simulink model "lead_acid_battery_estim"  (R2014a)
settings: Solver=ode15s  StartTime=0.0  StopTime=14787  RelTol=1e-3
PreLoadFcn:
  | ssc_lead_acid_battery_ini
  | load Measured_DATA
PostLoadFcn:
  | open_system([bdroot '/Orig. Values']);
  | warning off Simulink:blocks:MatchingFromNotFound
  | warning off Simulink:Engine:MdlFileShadowedByFile
undefined symbols (not defined in the file): Kt, Kt_Temps, sigbuilder_block, theta_f, theta_init
libraries: fl_lib x15, nesl_utility x6, LeadAcidBattery_lib x6
Description:
  | Lead-acid battery
  | 
  | This demo implements a model of a lead-acid battery cell using the Simscape
  | language to implement the nonlinear equations of the equivalent circuit
  | components. In this way, as opposed to modeling entirely in Simulink, the
  | connection between model components and the defining physical equations is
  | more easily understood. For the defining equations and their validation,
  | see Jackey, R. "A Simple, Effective Lead-Acid Battery Modeling Process for
  | Electrical System Component Selection",  SAE World Congress & Exhibition,
  | April 2007, ref. 2007-01-0778.
  | 
  | In this simulation, initially the battery is discharged at a constant current of 10A.
  | The battery is then recharged at a constant 10A back to the initial state of
  | charge. A simple thermal model is used to model battery temperature. It is
  | assumed that cooling is primarily via convection, and that heating is primarily
  | from battery internal resistance, R2. A standard 12 V lead-acid battery can
  | be modeled by connecting six copies of the 2V battery cell block in series.
  | Copyright 2014 The MathWorks, Inc.
settings Model: Creator=rhyde  LastModifiedBy=psanghvi
settings DataIOCC: ExternalInput=[Input_time, Input_Current_DATA]  LoadExternalInput=on  SignalLoggingSaveFormat=ModelDataLogs
settings OptimizationCC: ExpressionDepthLimit=2147483647
settings DebuggingCC: UnderspecifiedInitializationDetection=Classic  SolverPrmCheckMsg=none  FcnCallInpInsideContextMsg=UseLocalSettings  StateNameClashWarn=warning
settings GRTTargetCC: CombineOutputUpdateFcns=off  GRTInterface=on

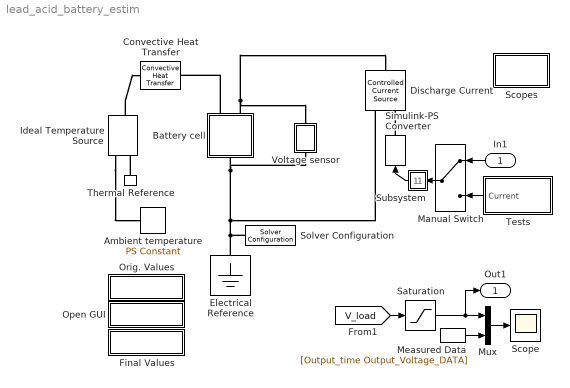
== system lead_acid_battery_estim ==
  In1 : Inport
  Ambient temperature : fl_lib/Physical Signals/Sources/PS Constant  constant=273+25
  Battery cell : Subsystem
      mask Display:
      | image(imread('battery.jpg'))
      | color('red')
      | port_label('LConn',1,'H')
      | port_label('LConn',2,'+')
      | port_label('RConn',1,'-')
  Convective Heat Transfer : fl_lib/Thermal/Thermal Elements/Convective Heat Transfer  area=Area m^2  heat_tr_coeff=Rtheta W/(m^2 * K)  Q_specify=off  Q_priority=High  Q=0 J/s  T_specify=off  T_priority=High  T=0 K
  Discharge Current : fl_lib/Electrical/Electrical Sources/Controlled Current Source
  Electrical Reference : fl_lib/Electrical/Electrical Elements/Electrical Reference
  Final Values : Subsystem
      settings: OpenFcn=load Battery_Param_Values_FINAL;
      mask Display: disp('Final Values')
  Ideal Temperature Source : fl_lib/Thermal/Thermal Sources/Ideal Temperature Source
  Manual Switch : ManualSwitch
  Measured Data : FromWorkspace  VariableName=[Output_time Output_Voltage_DATA]  SampleTime=0
  Mux : Mux  Inputs=2
  Open GUI : Subsystem
      settings: OpenFcn=speload('battery_estim', 'Project - lead_acid_battery_estim', 'Discharge Estimation');
      mask Display: disp('Open Tool')
  Orig. Values : Subsystem
      settings: OpenFcn=load Battery_Param_Values_START;
      mask Display: disp('Start Values')
  Saturation : Saturate  UpperLimit=3  LowerLimit=0
  Scope : Scope
      settings: TimeRange=15000  YMin=1.8  YMax=2.25  SaveName=Battery_DATA
  Scopes : Subsystem
  Simulink-PS Converter : nesl_utility/Simulink-PS Converter  PhysicalDomain=network_engine_domain  SubClassName=ps_input  LeftPortType=input  RightPortType=output  PseudoPeriodic=off  Frequencies=[]  NoiseDistribution=none  NoiseParameters=[]  Unit=A  AffineConversion=off  InputFiltering=off  SimscapeFilterOrder=1  InputFilterTimeConstant=.001  UdotUserProvided=0
  Solver Configuration : nesl_utility/Solver Configuration  PhysicalDomain=network_engine_domain  SubClassName=solver  LeftPortType=input  RightPortType=generic  Accelerate=off  Tones=[]  Harmonics=[]  SimulateNoise=off  Profile=off  UseLocalSampling=off  EnableSwitchedLinearOptims=on  FrequencyDomain=off  UseCCode=off  RelTol=0.001  AbsTol=1e-06  MinStep=1e-09  ToWorkspace=off  DoDC=off  ResidualTolerance=1e-9  UseLocalSolver=off  LocalSolverChoice=NE_BACKWARD_EULER_ADVANCER  LocalSolverSampleTime=.001  DoFixedCost=off  MaxNonlinIter=12  MaxModeIter=2  LinearAlgebra=Sparse  DelaysMemoryBudget=1024  AutomaticFiltering=on  FilteringTimeConstant=0.001
  Subsystem : Subsystem
      mask Display: disp('i')
  Tests : Subsystem  Tag=STV Subsys  LoadFcn=sigbuilder_block('load');  StartFcn=sigbuilder_block('start');  StopFcn=sigbuilder_block('stop');  ClipboardFcn=sigbuilder_block('clipboard');  mask(Sigbuilder block){}
      mask help: Sigbuilder GUI
      mask init:
      | if ~strcmp(get_param(bdroot(gcbh),'SimulationStatus'),'stopped') tuvar = sigbuilder_block('maskInit'); end
      settings: CopyFcn=sigbuilder_block('copy');  DeleteFcn=sigbuilder_block('delete');  ModelCloseFcn=sigbuilder_block('modelClose');  PreSaveFcn=sigbuilder_block('preSave');  PauseFcn=sigbuilder_block('pause')  ContinueFcn=sigbuilder_block('continue')  NameChangeFcn=sigbuilder_block('namechange');  OpenFcn=sigbuilder_block('open',[96 372 620.25 399.75 ]);  CloseFcn=sigbuilder_block('close');
      mask Display: plot(0,0,100,100,[10,10,40,40,10],[80,20,20,80,80],[40,10],[50,50], [40,27,10],[65,72,56],[40,25,25,10],[28,28,43,43]);
  Thermal Reference : fl_lib/Thermal/Thermal Elements/Thermal Reference
  Voltage sensor : Subsystem
  Out1 : Outport
  wires:
  [V_load] -> Saturation/1
  Saturation/1 -> Out1/1, Mux/1
  Mux/1 -> Scope/1
  Measured Data/1 -> Mux/2
  In1/1 -> Manual Switch/1
  Tests/1(Current) -> Manual Switch/2
  Manual Switch/1 -> Subsystem/1(In1)
  Subsystem/1(Out1) -> Simulink-PS Converter/1
  connections:
  Electrical Reference/LConn1 -- Voltage sensor/RConn1 -- Battery cell/RConn1 -- Discharge Current/RConn2 -- Solver Configuration/RConn1
  Discharge Current/LConn1 -- Voltage sensor/LConn1 -- Battery cell/LConn2
  Thermal Reference/LConn1 -- Ideal Temperature Source/RConn2
  Ideal Temperature Source/LConn1 -- Convective Heat Transfer/LConn1
  Ideal Temperature Source/RConn1 -- Ambient temperature/RConn1
  Battery cell/LConn1 -- Convective Heat Transfer/RConn1
  Simulink-PS Converter/RConn1 -- Discharge Current/RConn1

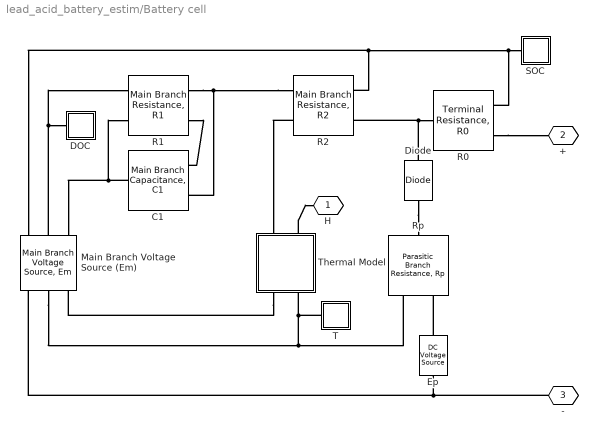
== system lead_acid_battery_estim/Battery cell ==
  " DOC " : Subsystem
  " SOC " : Subsystem
  C1 : LeadAcidBattery_lib/Main Branch Capacitance, C1  Tau1=Tau1 s  Cmin=1e-5 F  i_specify=off  i_priority=High  i=1 A  Q_specify=off  Q_priority=High  Q=0 V*F
  Diode : fl_lib/Electrical/Electrical Elements/Diode  Vf=0.6 V  Ron=0.3 Ohm  Goff=1e-08 1/Ohm  i_specify=off  i_priority=High  i=0 A  v_specify=off  v_priority=High  v=0 V
  Ep : fl_lib/Electrical/Electrical Sources/DC Voltage Source  v0=Ep V
  Main Branch Voltage Source (Em) : LeadAcidBattery_lib/Main Branch Voltage Source, Em  Em0=Emo V  Ke=Ke V/K  Kc=Kc  C0=Costar s*A  Istar=Istar A  delta=delta  Tau1=Tau1 s  Qinit=Qe_init s*A  i_specify=off  i_priority=High  i=0 A  Iavg_specify=off  Iavg_priority=High  Iavg=0 A  Qe_specify=off  Qe_priority=High  Qe=0 s*A
  R0 : LeadAcidBattery_lib/Terminal Resistance, R0  R00=Roo Ohm  A0=Ao  i_specify=off  i_priority=High  i=0 A
  R1 : LeadAcidBattery_lib/Main Branch Resistance, R1  R10=R10 Ohm  DOC_min=1e-006  i_specify=off  i_priority=High  i=0 A
  R2 : LeadAcidBattery_lib/Main Branch Resistance, R2  R20=R20 Ohm  A21=A21  A22=A22  Istar=Istar A  i_specify=off  i_priority=High  i=0 A
  Rp : LeadAcidBattery_lib/Parasitic Branch Resistance, Rp  Gp0=Gpo 1/Ohm  Vp0=Vpo V  Ap=Ap  Tf=theta_f C  i_specify=off  i_priority=High  i=0 A
  T : Subsystem
  Thermal Model : Subsystem
  H : PMIOPort  Tag=PMCPort  Port=1  Side=Left
  + : PMIOPort  Tag=PMCPort  Port=2  Side=Left
  - : PMIOPort  Tag=PMCPort  Port=3  Side=Right
  connections:
  T/LConn1 -- Thermal Model/RConn2 -- Rp/RConn1 -- Main Branch Voltage Source (Em)/RConn2
  R0/LConn2 -- +/RConn1
  Main Branch Voltage Source (Em)/LConn2 -- R1/RConn1 -- " DOC "/LConn1
  C1/RConn1 -- R1/RConn2 -- Main Branch Voltage Source (Em)/LConn3
  R2/RConn1 -- C1/LConn2 -- R1/LConn1
  R1/LConn2 -- C1/LConn1
  Main Branch Voltage Source (Em)/LConn1 -- R2/LConn1 -- R0/LConn1 -- " SOC "/LConn1
  Thermal Model/LConn2 -- H/RConn1
  Ep/LConn1 -- Rp/RConn2
  Diode/RConn1 -- Rp/LConn1
  Thermal Model/RConn1 -- Main Branch Voltage Source (Em)/RConn3
  Main Branch Voltage Source (Em)/RConn1 -- Ep/RConn1 -- -/RConn1
  R2/RConn2 -- Thermal Model/LConn1
  R2/LConn2 -- R0/RConn1 -- Diode/LConn1

== system lead_acid_battery_estim/Final Values ==

== system lead_acid_battery_estim/Open GUI ==

== system lead_acid_battery_estim/Orig. Values ==

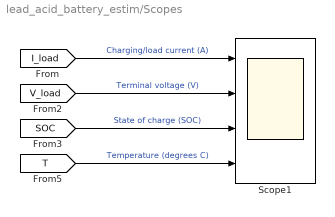
== system lead_acid_battery_estim/Scopes ==
  Scope1 : Scope  NumInputPorts=4
      settings: TimeRange=15000  YMin=-10~1.8~0~24  YMax=-0~2~1~26
  wires:
  [V_load] -> Scope1/2  "Terminal voltage (V)"
  [SOC] -> Scope1/3  "State of charge (SOC)"
  [T] -> Scope1/4  "Temperature (degrees C)"
  [I_load] -> Scope1/1  "Charging/load current (A)"

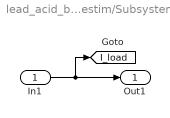
== system lead_acid_battery_estim/Subsystem ==
  In1 : Inport
  Out1 : Outport
  tag scope: I_load=global
  wires:
  In1/1 -> [I_load], Out1/1

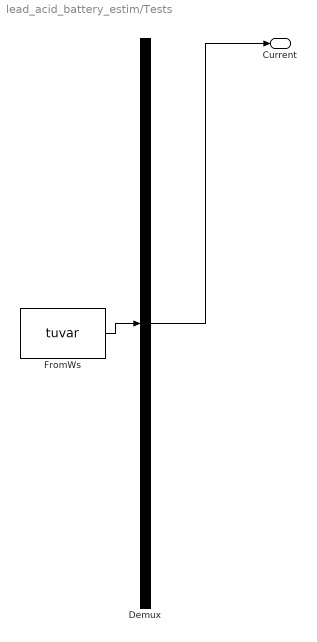
== system lead_acid_battery_estim/Tests ==
  Demux : Demux  Tag=STV Demux  Outputs=1
  FromWs : FromWorkspace  Tag=STV FromWs  VariableName=tuvar  SampleTime=0
      SigBuilderData=|
      | common.afterFinalStr = 'Extrapolate'
      | common.sampleTime = 0
      | dataSet(1).timeRange = [0 36000]
      | dataSet(1).name = 'Dynamic'
      | dataSet(2).timeRange = [0 36000]
      | dataSet(2).name = 'Charge Cycle'
      | dataSet(3).timeRange = [0 36000]
      | dataSet(3).name = 'Square'
      | sbobj.Groups(1).Name = 'Dynamic'
      | sbobj.Groups(1).Signals.Name = 'Current'
      | sbobj.Groups(1).Signals.XData = [0 60 120 180 240 300 360 420 480 540 600 660 ... (607 elements, 1x607)]
      | sbobj.Groups(1).Signals.YData = [-4.32564811528 -16.6558437824 1.25332306475 2.87676420359 -11.4647135068 11.9091546564 11.8916420165 -0.376332765933 3.27292361409 1.74639142821 -1.86708577681 7.25790548293 ... (607 elements, 1x607)]
      | sbobj.Groups(2).Name = 'Charge Cycle'
      | sbobj.Groups(2).Signals.Name = 'Current'
      | sbobj.Groups(2).Signals.XData = [0 1000 1000 12585 12595 18400 18400 28090 35015 36000]
      | sbobj.Groups(2).Signals.YData = [0 0 -10 -10 0 0 10 10 0 0]
      | sbobj.Groups(3).Name = 'Square'
      | sbobj.Groups(3).Signals.Name = 'Current'
      | sbobj.Groups(3).Signals.XData = [0 3600 3600 5400 5400 7200 7200 9000 9000 10800 10800 12600 12600 14400 14400 16200 16200 18000 18000 19800 19800 21600 21600 23400 23400 25200 25200 27000 27000 28800 28800 30600 30600 32400 32400 34200 34200 36000]
      | sbobj.Groups(3).Signals.YData = [-20 -20 0 0 20 20 -20 -20 20 20 -20 -20 20 20 -20 -20 20 20 -20 -20 20 20 -20 -20 20 20 -20 -20 20 20 -20 -20 20 20 -20 -20 20 20]
  Current : Outport  Tag=STV Outport
  wires:
  Demux/1 -> Current/1
  FromWs/1 -> Demux/1

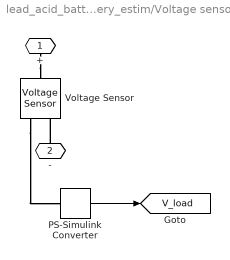
== system lead_acid_battery_estim/Voltage sensor ==
  PS-Simulink Converter : nesl_utility/PS-Simulink Converter  PhysicalDomain=network_engine_domain  SubClassName=ps_output  LeftPortType=input  RightPortType=output  PseudoPeriodic=off  Frequencies=[]  Unit=V  AffineConversion=off
  Voltage Sensor : fl_lib/Electrical/Electrical Sensors/Voltage Sensor
  + : PMIOPort  Port=1  Side=Left
  - : PMIOPort  Port=2  Side=Right
  tag scope: V_load=global
  wires:
  PS-Simulink Converter/1 -> [V_load]
  connections:
  Voltage Sensor/RConn1 -- PS-Simulink Converter/LConn1
  +/RConn1 -- Voltage Sensor/LConn1
  -/RConn1 -- Voltage Sensor/RConn2

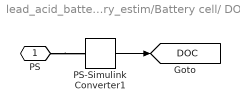
== system lead_acid_battery_estim/Battery cell/ DOC  ==
  PS-Simulink Converter1 : nesl_utility/PS-Simulink Converter  PhysicalDomain=network_engine_domain  SubClassName=ps_output  LeftPortType=input  RightPortType=output  PseudoPeriodic=off  Frequencies=[]  Unit=1  AffineConversion=off
  PS : PMIOPort  Port=1  Side=Left
  tag scope: DOC=global
  wires:
  PS-Simulink Converter1/1 -> [DOC]
  connections:
  PS/RConn1 -- PS-Simulink Converter1/LConn1

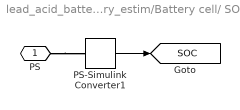
== system lead_acid_battery_estim/Battery cell/ SOC  ==
  PS-Simulink Converter1 : nesl_utility/PS-Simulink Converter  PhysicalDomain=network_engine_domain  SubClassName=ps_output  LeftPortType=input  RightPortType=output  PseudoPeriodic=off  Frequencies=[]  Unit=1  AffineConversion=off
  PS : PMIOPort  Port=1  Side=Left
  tag scope: SOC=global
  wires:
  PS-Simulink Converter1/1 -> [SOC]
  connections:
  PS/RConn1 -- PS-Simulink Converter1/LConn1

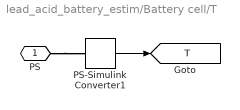
== system lead_acid_battery_estim/Battery cell/T ==
  PS-Simulink Converter1 : nesl_utility/PS-Simulink Converter  PhysicalDomain=network_engine_domain  SubClassName=ps_output  LeftPortType=input  RightPortType=output  PseudoPeriodic=off  Frequencies=[]  Unit=C  AffineConversion=on
  PS : PMIOPort  Port=1  Side=Left
  tag scope: T=global
  wires:
  PS-Simulink Converter1/1 -> [T]
  connections:
  PS/RConn1 -- PS-Simulink Converter1/LConn1

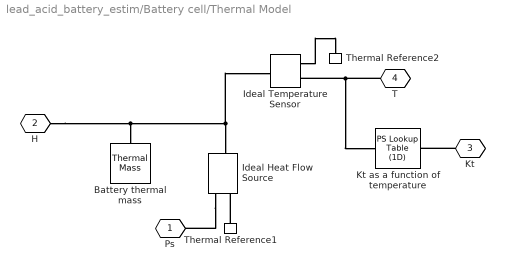
== system lead_acid_battery_estim/Battery cell/Thermal Model ==
  Battery thermal mass : fl_lib/Thermal/Thermal Elements/Thermal Mass  mass=1 kg  sp_heat=Ctheta J/kg/K  Q_specify=off  Q_priority=High  Q=0 J/s  T_specify=on  T_priority=High  T=theta_init+273 K
  Ideal Temperature Sensor : fl_lib/Thermal/Thermal Sensors/Ideal Temperature Sensor
  Ideal Heat Flow Source : fl_lib/Thermal/Thermal Sources/Ideal Heat Flow Source
  Kt as a function of temperature : fl_lib/Physical Signals/Lookup Tables/PS Lookup Table (1D)  x_t=[theta_f, Kt_Temps]+273  y_t=[0 Kt]  interp_method=1  extrap_method=1
  Thermal Reference1 : fl_lib/Thermal/Thermal Elements/Thermal Reference
  Thermal Reference2 : fl_lib/Thermal/Thermal Elements/Thermal Reference
  Ps : PMIOPort  Tag=PMCPort  Port=1  Side=Left
  H : PMIOPort  Tag=PMCPort  Port=2  Side=Left
  Kt : PMIOPort  Tag=PMCPort  Port=3  Side=Right
  T : PMIOPort  Tag=PMCPort  Port=4  Side=Right
  connections:
  Ideal Temperature Sensor/RConn1 -- Thermal Reference2/LConn1
  Ideal Temperature Sensor/RConn2 -- Kt as a function of temperature/LConn1 -- T/RConn1
  Thermal Reference1/LConn1 -- Ideal Heat Flow Source/RConn2
  H/RConn1 -- Ideal Temperature Sensor/LConn1 -- Ideal Heat Flow Source/LConn1 -- Battery thermal mass/LConn1
  Kt/RConn1 -- Kt as a function of temperature/RConn1
  Ideal Heat Flow Source/RConn1 -- Ps/RConn1
